simulink model "Drone_dynamic_controle_PID"  (R2024b)
settings: Solver=VariableStepAuto  StartTime=0.0  StopTime=20  RelTol=1e-3
values from neighbouring files (symbols this model uses):
  b = 4*1e-4    (= 0.0004)    [Drone_parameters.m]    (also in Quadcopter.m = 1e-06; drone_dynamics.m = 1e-06)
  g = 9.81    [Drone_parameters.m]    (also in Quadcopter.m; drone_dynamics.m)
  Ix = 0.02    [Drone_parameters.m]    (also in drone_dynamics.m)
  Iy = 0.02    [Drone_parameters.m]    (also in drone_dynamics.m)
  Iz = 0.04    [Drone_parameters.m]    (also in drone_dynamics.m)
  kf = T*0.7/w^2 * 0.8    (= 6.88114119063e-05)    [Drone_parameters.m]
  m = 1.2    [Drone_parameters.m]    (also in Quadcopter.m = 1; drone_dynamics.m)
  w_max = 2*3.14*n_max/60    (= 3061.60466667)    [Drone_parameters.m]
undefined symbols (not defined in the file or in its folder): a, balljoint_offset, k_cmd2rad, Kd_phi, Kd_psi, Kd_th, Kd_z, Ki_phi, Ki_psi, Ki_th, Ki_z, Kp_phi, Kp_psi, Kp_th, Kp_z, N_d, omega_max, omega_min, PID_LIMIT, PID_LIMIT_Z, s_max, s_min, SPEED_OFFSET, tau_m, tau_s, wmax
libraries: slpidlib x8
settings Model: Creator=lolme  LastModifiedBy=Rogul

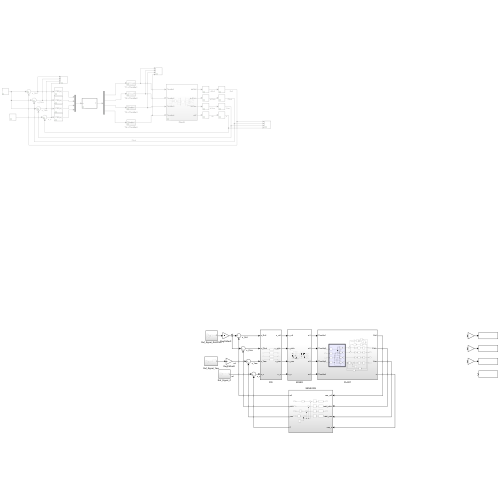
[thumbnail: Simulink's stored preview of the top-level diagram]
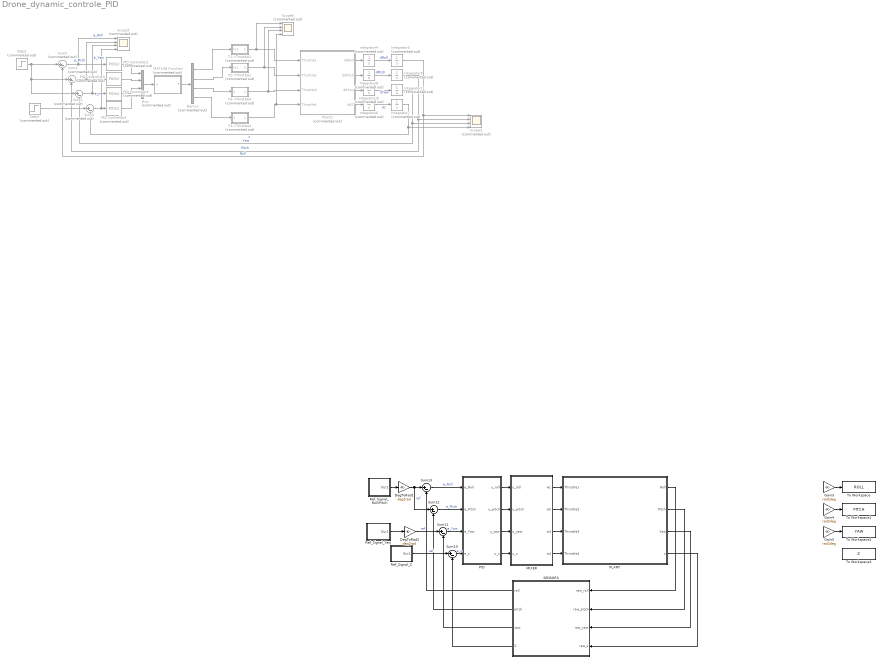
== system Drone_dynamic_controle_PID ==
  DegToRad1 : Gain  Gain=deg2rad
  DegToRad2 : Gain  Gain=deg2rad
  Demux : Demux  Commented=on
  Gain3 : Gain  Gain=rad2deg
  Gain4 : Gain  Gain=rad2deg
  Gain5 : Gain  Gain=rad2deg
  Integrator{4..11} (8 alike) : Integrator  Commented=on
  MATLAB Function : MATLAB Function  Commented=on  TreatAsAtomicUnit=on
  MIXER : Subsystem
  Mux : Mux  Commented=on
  PID : Subsystem
  PID Controller2 : slpidlib/PID Controller  Commented=on  Controller=PID  Form=Parallel  TimeDomain=Continuous-time  UseExternalTs=off  SampleTime=-1  IntegratorMethod=Forward Euler  FilterMethod=Forward Euler  ControllerParametersSource=internal  P=1.5  I=0.05  UseKiTs=off  D=0.3  UseExternalDerivativeSource=off  N=100  UseFilter=on  TunerSelectOption=Transfer Function Based (PID Tuner App)  InitialConditionSource=internal  InitialConditionForIntegrator=0  InitialConditionForFilter=0  DifferentiatorICPrevScaledInput=0  ExternalReset=none  TrackingMode=off  Kt=1  LimitOutput=off  SatLimitsSource=internal  UpperSaturationLimit=inf  LowerSaturationLimit=-inf  LinearizeAsGain=on  AntiWindupMode=none  Kb=1  LimitIntegrator=off  UpperIntegratorSaturationLimit=inf  LowerIntegratorSaturationLimit=-inf  POutMin=[]  POutMax=[]  IOutMin=[]  IOutMax=[]  DOutMin=[]  DOutMax=[]  NOutMin=[]  NOutMax=[]  SumOutMin=[]  SumOutMax=[]  SaturationOutMin=[]  SaturationOutMax=[]  PParamMin=[]  PParamMax=[]  IParamMin=[]  IParamMax=[]  DParamMin=[]  DParamMax=[]  NParamMin=[]  NParamMax=[]  KbParamMin=[]  KbParamMax=[]  KtParamMin=[]  KtParamMax=[]  KbOutMin=[]  KbOutMax=[]  KtOutMin=[]  KtOutMax=[]  IntegratorOutMin=[]  IntegratorOutMax=[]  FilterOutMin=[]  FilterOutMax=[]  SumI1OutMin=[]  SumI1OutMax=[]  SumI2OutMin=[]  SumI2OutMax=[]  SumI3OutMin=[]  SumI3OutMax=[]  SumI4OutMin=[]  SumI4OutMax=[]  SumDOutMin=[]  SumDOutMax=[]  DifferentiatorOutMin=[]  DifferentiatorOutMax=[]  FilterDiffOutCoefMin=[]  FilterDiffOutCoefMax=[]  ReciprocalOutMin=[]  ReciprocalOutMax=[]  SumDenOutMin=[]  SumDenOutMax=[]  SumNumOutMin=[]  SumNumOutMax=[]  DivideOutMin=[]  DivideOutMax=[]  UdiffTsProdOutMin=[]  UdiffTsProdOutMax=[]  NTsProdOutMin=[]  NTsProdOutMax=[]  UintegralTsProdOutMin=[]  UintegralTsProdOutMax=[]  UngainTsProdOutMin=[]  UngainTsProdOutMax=[]  ClampingZeroOutDataTypeStr=Inherit: Inherit via back propagation  ClampingZeroOutMin=[]  ClampingZeroOutMax=[]  FilterDenConstantOutDataTypeStr=Inherit: Inherit via back propagation  FilterDenConstantOutMin=[]  FilterDenConstantOutMax=[]  PCopyOutDataTypeStr=Inherit: Inherit via back propagation  PCopyOutMin=[]  PCopyOutMax=[]  NCopyOutDataTypeStr=Inherit: Inherit via back propagation  NCopyOutMin=[]  NCopyOutMax=[]  IntegratorContinuousStateAttributes=''  IntegratorStateMustResolveToSignalObject=off  IntegratorRTWStateStorageClass=Auto  FilterContinuousStateAttributes=''  FilterStateMustResolveToSignalObject=off  FilterRTWStateStorageClass=Auto  ParallelPVariant=InternalParameters  IdealPVariant=Disabled  IVariant=InternalParameters  DVariant=InternalParameters  IntegratorVariant=Continuous  SatVariant=Disabled  AWVariant=Passthrough  PCopyVariant=Disabled  TRVariant=Disabled  FdbkBlocksVariant=Forward  IdealPFdbkVariant=Disabled  SatFdbkVariant=Disabled  DerivativeFilterVariant=ContFilter  NVariant=InternalParameters  NCopyVariant=Disabled  FilterICVariant=InternalICsFilter  IntegratorICVariant=InternalICs  ExternalResetVariant=Disabled  TRSumVariant=Passthrough  SumFdbkVariant=Disabled  SumVariant=Sum_PID  TsampFilterVariant=InternalTs  TsampNgainVariant=Passthrough  TsampIntegralVariant=Disabled_SignalSpec  ExternalSaturationOutDataTypeStr=Inherit: Same as second input  DerivativeSourceVariant=ErrorSignal  PreIntVariant=InternalPreInt
  PID Controller3 : slpidlib/PID Controller  Commented=on  Controller=PID  Form=Parallel  TimeDomain=Continuous-time  UseExternalTs=off  SampleTime=-1  IntegratorMethod=Forward Euler  FilterMethod=Forward Euler  ControllerParametersSource=internal  P=1.5  I=0.05  UseKiTs=off  D=0.3  UseExternalDerivativeSource=off  N=100  UseFilter=on  TunerSelectOption=Transfer Function Based (PID Tuner App)  InitialConditionSource=internal  InitialConditionForIntegrator=0  InitialConditionForFilter=0  DifferentiatorICPrevScaledInput=0  ExternalReset=none  TrackingMode=off  Kt=1  LimitOutput=off  SatLimitsSource=internal  UpperSaturationLimit=inf  LowerSaturationLimit=-inf  LinearizeAsGain=on  AntiWindupMode=none  Kb=1  LimitIntegrator=off  UpperIntegratorSaturationLimit=inf  LowerIntegratorSaturationLimit=-inf  POutMin=[]  POutMax=[]  IOutMin=[]  IOutMax=[]  DOutMin=[]  DOutMax=[]  NOutMin=[]  NOutMax=[]  SumOutMin=[]  SumOutMax=[]  SaturationOutMin=[]  SaturationOutMax=[]  PParamMin=[]  PParamMax=[]  IParamMin=[]  IParamMax=[]  DParamMin=[]  DParamMax=[]  NParamMin=[]  NParamMax=[]  KbParamMin=[]  KbParamMax=[]  KtParamMin=[]  KtParamMax=[]  KbOutMin=[]  KbOutMax=[]  KtOutMin=[]  KtOutMax=[]  IntegratorOutMin=[]  IntegratorOutMax=[]  FilterOutMin=[]  FilterOutMax=[]  SumI1OutMin=[]  SumI1OutMax=[]  SumI2OutMin=[]  SumI2OutMax=[]  SumI3OutMin=[]  SumI3OutMax=[]  SumI4OutMin=[]  SumI4OutMax=[]  SumDOutMin=[]  SumDOutMax=[]  DifferentiatorOutMin=[]  DifferentiatorOutMax=[]  FilterDiffOutCoefMin=[]  FilterDiffOutCoefMax=[]  ReciprocalOutMin=[]  ReciprocalOutMax=[]  SumDenOutMin=[]  SumDenOutMax=[]  SumNumOutMin=[]  SumNumOutMax=[]  DivideOutMin=[]  DivideOutMax=[]  UdiffTsProdOutMin=[]  UdiffTsProdOutMax=[]  NTsProdOutMin=[]  NTsProdOutMax=[]  UintegralTsProdOutMin=[]  UintegralTsProdOutMax=[]  UngainTsProdOutMin=[]  UngainTsProdOutMax=[]  ClampingZeroOutDataTypeStr=Inherit: Inherit via back propagation  ClampingZeroOutMin=[]  ClampingZeroOutMax=[]  FilterDenConstantOutDataTypeStr=Inherit: Inherit via back propagation  FilterDenConstantOutMin=[]  FilterDenConstantOutMax=[]  PCopyOutDataTypeStr=Inherit: Inherit via back propagation  PCopyOutMin=[]  PCopyOutMax=[]  NCopyOutDataTypeStr=Inherit: Inherit via back propagation  NCopyOutMin=[]  NCopyOutMax=[]  IntegratorContinuousStateAttributes=''  IntegratorStateMustResolveToSignalObject=off  IntegratorRTWStateStorageClass=Auto  FilterContinuousStateAttributes=''  FilterStateMustResolveToSignalObject=off  FilterRTWStateStorageClass=Auto  ParallelPVariant=InternalParameters  IdealPVariant=Disabled  IVariant=InternalParameters  DVariant=InternalParameters  IntegratorVariant=Continuous  SatVariant=Disabled  AWVariant=Passthrough  PCopyVariant=Disabled  TRVariant=Disabled  FdbkBlocksVariant=Forward  IdealPFdbkVariant=Disabled  SatFdbkVariant=Disabled  DerivativeFilterVariant=ContFilter  NVariant=InternalParameters  NCopyVariant=Disabled  FilterICVariant=InternalICsFilter  IntegratorICVariant=InternalICs  ExternalResetVariant=Disabled  TRSumVariant=Passthrough  SumFdbkVariant=Disabled  SumVariant=Sum_PID  TsampFilterVariant=InternalTs  TsampNgainVariant=Passthrough  TsampIntegralVariant=Disabled_SignalSpec  ExternalSaturationOutDataTypeStr=Inherit: Same as second input  DerivativeSourceVariant=ErrorSignal  PreIntVariant=InternalPreInt
  PID Controller4 : slpidlib/PID Controller  Commented=on  Controller=PID  Form=Parallel  TimeDomain=Continuous-time  UseExternalTs=off  SampleTime=-1  IntegratorMethod=Forward Euler  FilterMethod=Forward Euler  ControllerParametersSource=internal  P=1.5  I=0.05  UseKiTs=off  D=0.3  UseExternalDerivativeSource=off  N=100  UseFilter=on  TunerSelectOption=Transfer Function Based (PID Tuner App)  InitialConditionSource=internal  InitialConditionForIntegrator=0  InitialConditionForFilter=0  DifferentiatorICPrevScaledInput=0  ExternalReset=none  TrackingMode=off  Kt=1  LimitOutput=off  SatLimitsSource=internal  UpperSaturationLimit=inf  LowerSaturationLimit=-inf  LinearizeAsGain=on  AntiWindupMode=none  Kb=1  LimitIntegrator=off  UpperIntegratorSaturationLimit=inf  LowerIntegratorSaturationLimit=-inf  POutMin=[]  POutMax=[]  IOutMin=[]  IOutMax=[]  DOutMin=[]  DOutMax=[]  NOutMin=[]  NOutMax=[]  SumOutMin=[]  SumOutMax=[]  SaturationOutMin=[]  SaturationOutMax=[]  PParamMin=[]  PParamMax=[]  IParamMin=[]  IParamMax=[]  DParamMin=[]  DParamMax=[]  NParamMin=[]  NParamMax=[]  KbParamMin=[]  KbParamMax=[]  KtParamMin=[]  KtParamMax=[]  KbOutMin=[]  KbOutMax=[]  KtOutMin=[]  KtOutMax=[]  IntegratorOutMin=[]  IntegratorOutMax=[]  FilterOutMin=[]  FilterOutMax=[]  SumI1OutMin=[]  SumI1OutMax=[]  SumI2OutMin=[]  SumI2OutMax=[]  SumI3OutMin=[]  SumI3OutMax=[]  SumI4OutMin=[]  SumI4OutMax=[]  SumDOutMin=[]  SumDOutMax=[]  DifferentiatorOutMin=[]  DifferentiatorOutMax=[]  FilterDiffOutCoefMin=[]  FilterDiffOutCoefMax=[]  ReciprocalOutMin=[]  ReciprocalOutMax=[]  SumDenOutMin=[]  SumDenOutMax=[]  SumNumOutMin=[]  SumNumOutMax=[]  DivideOutMin=[]  DivideOutMax=[]  UdiffTsProdOutMin=[]  UdiffTsProdOutMax=[]  NTsProdOutMin=[]  NTsProdOutMax=[]  UintegralTsProdOutMin=[]  UintegralTsProdOutMax=[]  UngainTsProdOutMin=[]  UngainTsProdOutMax=[]  ClampingZeroOutDataTypeStr=Inherit: Inherit via back propagation  ClampingZeroOutMin=[]  ClampingZeroOutMax=[]  FilterDenConstantOutDataTypeStr=Inherit: Inherit via back propagation  FilterDenConstantOutMin=[]  FilterDenConstantOutMax=[]  PCopyOutDataTypeStr=Inherit: Inherit via back propagation  PCopyOutMin=[]  PCopyOutMax=[]  NCopyOutDataTypeStr=Inherit: Inherit via back propagation  NCopyOutMin=[]  NCopyOutMax=[]  IntegratorContinuousStateAttributes=''  IntegratorStateMustResolveToSignalObject=off  IntegratorRTWStateStorageClass=Auto  FilterContinuousStateAttributes=''  FilterStateMustResolveToSignalObject=off  FilterRTWStateStorageClass=Auto  ParallelPVariant=InternalParameters  IdealPVariant=Disabled  IVariant=InternalParameters  DVariant=InternalParameters  IntegratorVariant=Continuous  SatVariant=Disabled  AWVariant=Passthrough  PCopyVariant=Disabled  TRVariant=Disabled  FdbkBlocksVariant=Forward  IdealPFdbkVariant=Disabled  SatFdbkVariant=Disabled  DerivativeFilterVariant=ContFilter  NVariant=InternalParameters  NCopyVariant=Disabled  FilterICVariant=InternalICsFilter  IntegratorICVariant=InternalICs  ExternalResetVariant=Disabled  TRSumVariant=Passthrough  SumFdbkVariant=Disabled  SumVariant=Sum_PID  TsampFilterVariant=InternalTs  TsampNgainVariant=Passthrough  TsampIntegralVariant=Disabled_SignalSpec  ExternalSaturationOutDataTypeStr=Inherit: Same as second input  DerivativeSourceVariant=ErrorSignal  PreIntVariant=InternalPreInt
  PID Controller5 : slpidlib/PID Controller  Commented=on  Controller=PID  Form=Parallel  TimeDomain=Continuous-time  UseExternalTs=off  SampleTime=-1  IntegratorMethod=Forward Euler  FilterMethod=Forward Euler  ControllerParametersSource=internal  P=20  I=5  UseKiTs=off  D=10  UseExternalDerivativeSource=off  N=100  UseFilter=on  TunerSelectOption=Transfer Function Based (PID Tuner App)  InitialConditionSource=internal  InitialConditionForIntegrator=0  InitialConditionForFilter=0  DifferentiatorICPrevScaledInput=0  ExternalReset=none  TrackingMode=off  Kt=1  LimitOutput=off  SatLimitsSource=internal  UpperSaturationLimit=inf  LowerSaturationLimit=-inf  LinearizeAsGain=on  AntiWindupMode=none  Kb=1  LimitIntegrator=off  UpperIntegratorSaturationLimit=inf  LowerIntegratorSaturationLimit=-inf  POutMin=[]  POutMax=[]  IOutMin=[]  IOutMax=[]  DOutMin=[]  DOutMax=[]  NOutMin=[]  NOutMax=[]  SumOutMin=[]  SumOutMax=[]  SaturationOutMin=[]  SaturationOutMax=[]  PParamMin=[]  PParamMax=[]  IParamMin=[]  IParamMax=[]  DParamMin=[]  DParamMax=[]  NParamMin=[]  NParamMax=[]  KbParamMin=[]  KbParamMax=[]  KtParamMin=[]  KtParamMax=[]  KbOutMin=[]  KbOutMax=[]  KtOutMin=[]  KtOutMax=[]  IntegratorOutMin=[]  IntegratorOutMax=[]  FilterOutMin=[]  FilterOutMax=[]  SumI1OutMin=[]  SumI1OutMax=[]  SumI2OutMin=[]  SumI2OutMax=[]  SumI3OutMin=[]  SumI3OutMax=[]  SumI4OutMin=[]  SumI4OutMax=[]  SumDOutMin=[]  SumDOutMax=[]  DifferentiatorOutMin=[]  DifferentiatorOutMax=[]  FilterDiffOutCoefMin=[]  FilterDiffOutCoefMax=[]  ReciprocalOutMin=[]  ReciprocalOutMax=[]  SumDenOutMin=[]  SumDenOutMax=[]  SumNumOutMin=[]  SumNumOutMax=[]  DivideOutMin=[]  DivideOutMax=[]  UdiffTsProdOutMin=[]  UdiffTsProdOutMax=[]  NTsProdOutMin=[]  NTsProdOutMax=[]  UintegralTsProdOutMin=[]  UintegralTsProdOutMax=[]  UngainTsProdOutMin=[]  UngainTsProdOutMax=[]  ClampingZeroOutDataTypeStr=Inherit: Inherit via back propagation  ClampingZeroOutMin=[]  ClampingZeroOutMax=[]  FilterDenConstantOutDataTypeStr=Inherit: Inherit via back propagation  FilterDenConstantOutMin=[]  FilterDenConstantOutMax=[]  PCopyOutDataTypeStr=Inherit: Inherit via back propagation  PCopyOutMin=[]  PCopyOutMax=[]  NCopyOutDataTypeStr=Inherit: Inherit via back propagation  NCopyOutMin=[]  NCopyOutMax=[]  IntegratorContinuousStateAttributes=''  IntegratorStateMustResolveToSignalObject=off  IntegratorRTWStateStorageClass=Auto  FilterContinuousStateAttributes=''  FilterStateMustResolveToSignalObject=off  FilterRTWStateStorageClass=Auto  ParallelPVariant=InternalParameters  IdealPVariant=Disabled  IVariant=InternalParameters  DVariant=InternalParameters  IntegratorVariant=Continuous  SatVariant=Disabled  AWVariant=Passthrough  PCopyVariant=Disabled  TRVariant=Disabled  FdbkBlocksVariant=Forward  IdealPFdbkVariant=Disabled  SatFdbkVariant=Disabled  DerivativeFilterVariant=ContFilter  NVariant=InternalParameters  NCopyVariant=Disabled  FilterICVariant=InternalICsFilter  IntegratorICVariant=InternalICs  ExternalResetVariant=Disabled  TRSumVariant=Passthrough  SumFdbkVariant=Disabled  SumVariant=Sum_PID  TsampFilterVariant=InternalTs  TsampNgainVariant=Passthrough  TsampIntegralVariant=Disabled_SignalSpec  ExternalSaturationOutDataTypeStr=Inherit: Same as second input  DerivativeSourceVariant=ErrorSignal  PreIntVariant=InternalPreInt
  PLANT : Subsystem
  Plant2 : Subsystem  Commented=on
  Ref_Signal_Roll/Pitch : Subsystem
  Ref_Signal_Yaw : Subsystem
  Ref_Signal_Z : Subsystem
  SENSORS : Subsystem
  Scope3 : Scope  Commented=on  NumInputPorts=4
  Scope5 : Scope  Commented=on  NumInputPorts=4
  Scope6 : Scope  Commented=on  NumInputPorts=4
  Step2 : Step  Commented=on  Time=5  Before=20  After=0  SampleTime=0
  Step3 : Step  Commented=on  Time=5  Before=10  After=20  SampleTime=0
  Sum{10..13} (4 alike) : Sum  Inputs=|+-
  Sum{2..5} (4 alike) : Sum  Commented=on  Inputs=|+-
  T1->Throttle1 : Subsystem  Commented=on
  T2->Throttle2 : Subsystem  Commented=on
  T3->Throttle3 : Subsystem  Commented=on
  T4->Throttle4 : Subsystem  Commented=on
  To Workspace : ToWorkspace  VariableName=ROLL  SaveFormat=Timeseries  SampleTime=0.01
      settings: Save2DSignal=2-D array (concatenate along first dimension)
  To Workspace1 : ToWorkspace  VariableName=PITCH  SaveFormat=Timeseries  SampleTime=0.01
      settings: Save2DSignal=2-D array (concatenate along first dimension)
  To Workspace2 : ToWorkspace  VariableName=YAW  SaveFormat=Timeseries  SampleTime=0.01
      settings: Save2DSignal=2-D array (concatenate along first dimension)
  To Workspace3 : ToWorkspace  VariableName=Z  SaveFormat=Timeseries  SampleTime=0.01
      settings: Save2DSignal=2-D array (concatenate along first dimension)
  wires:
  Integrator7/1 -> Scope3/4, Sum2/2  "z"
  Integrator4/1 -> Integrator5/1  "dRoll"
  Plant2/1(ddRoll) -> Integrator4/1
  Integrator6/1 -> Integrator7/1  "dz"
  Integrator5/1 -> Scope3/1, Sum5/2  "Roll"
  Plant2/4(ddZ) -> Integrator6/1
  Integrator9/1 -> Scope3/2, Sum4/2  "Pitch"
  Plant2/2(ddPitch) -> Integrator8/1
  Integrator8/1 -> Integrator9/1  "dPitch"
  Plant2/3(ddYaw) -> Integrator10/1
  Integrator10/1 -> Integrator11/1  "dYaw"
  Integrator11/1 -> Scope3/3, Sum3/2  "Yaw"
  Sum2/1 -> Scope5/4, PID Controller5/1  "e_z"
  Sum3/1 -> Scope5/3, PID Controller4/1  "e_Yaw"
  Sum4/1 -> Scope5/2, PID Controller3/1  "e_Pitch"
  Sum5/1 -> Scope5/1, PID Controller2/1  "e_Roll"
  Step2/1 -> Sum3/1, Sum4/1, Sum5/1
  Step3/1 -> Sum2/1
  PID Controller2/1 -> Mux/1
  PID Controller3/1 -> Mux/2
  PID Controller4/1 -> Mux/3
  PID Controller5/1 -> Mux/4
  Mux/1 -> MATLAB Function/1(u)
  MATLAB Function/1(T) -> Demux/1
  Demux/1 -> T1->Throttle1/1(In1)
  T2->Throttle2/1(1) -> Scope6/2, Plant2/2(Throttle2)
  Demux/2 -> T2->Throttle2/1(In1)
  T3->Throttle3/1(Throttle1) -> Scope6/3, Plant2/3(Throttle3)
  Demux/3 -> T3->Throttle3/1(In1)
  T4->Throttle4/1(Throttle1) -> Scope6/4, Plant2/4(Throttle4)
  Demux/4 -> T4->Throttle4/1(In1)
  T1->Throttle1/1(1) -> Scope6/1, Plant2/1(Throttle1)
  Ref_Signal_Roll/Pitch/1(Out1) -> DegToRad1/1
  Ref_Signal_Yaw/1(Out1) -> DegToRad2/1
  Ref_Signal_Z/1(Out1) -> Sum10/1  "ref"
  DegToRad1/1 -> Sum13/1, Sum12/1  "ref"
  DegToRad2/1 -> Sum11/1  "ref"
  MIXER/1(w1) -> PLANT/1(Throttle1)
  MIXER/2(w2) -> PLANT/2(Throttle2)
  MIXER/3(w3) -> PLANT/3(Throttle3)
  MIXER/4(w4) -> PLANT/4(Throttle4)
  Gain3/1 -> To Workspace/1
  Gain4/1 -> To Workspace1/1
  Gain5/1 -> To Workspace2/1
  Sum13/1 -> PID/1(e_Roll)  "e_Roll"
  Sum12/1 -> PID/2(e_Pitch)  "e_Pitch"
  Sum11/1 -> PID/3(e_Yaw)  "e_Yaw"
  Sum10/1 -> PID/4(e_z)  "e_z"
  PID/1(u_roll) -> MIXER/1(u_roll)
  PID/2(u_pitch) -> MIXER/2(u_pitch)
  PID/3(u_yaw) -> MIXER/3(u_yaw)
  PID/4(u_z) -> MIXER/4(u_z)
  PLANT/1(Roll) -> SENSORS/1(raw_roll)
  PLANT/2(Pitch) -> SENSORS/2(raw_pitch)
  PLANT/3(Yaw) -> SENSORS/3(raw_yaw)
  PLANT/4(z) -> SENSORS/4(raw_z)
  SENSORS/1(roll) -> Sum13/2
  SENSORS/2(pitch) -> Sum12/2
  SENSORS/4(Z) -> Sum10/2
  SENSORS/3(yaw) -> Sum11/2

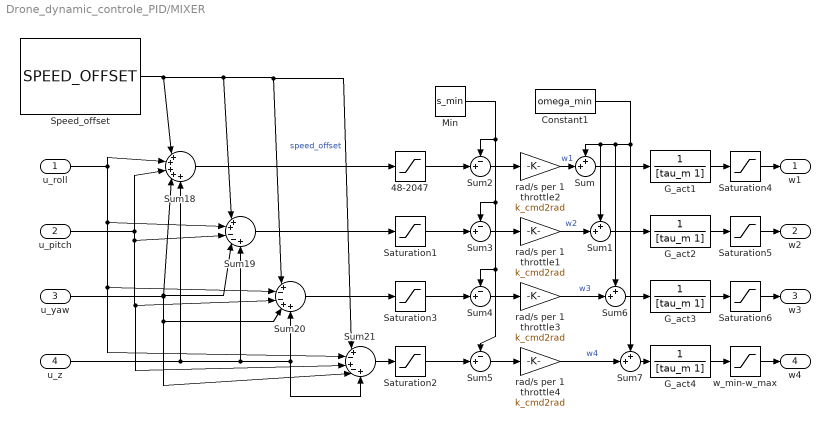
== system Drone_dynamic_controle_PID/MIXER ==
  u_roll : Inport
  u_pitch : Inport  Port=2
  u_yaw : Inport  Port=3
  u_z : Inport  Port=4
  48-2047 : Saturate  UpperLimit=s_max  LowerLimit=s_min
  Constant1 : Constant  Value=omega_min
  G_act{1..4} (4 alike) : TransferFcn  Denominator=[tau_m 1]
  Min : Constant  Value=s_min
  Saturation1 : Saturate  UpperLimit=s_max  LowerLimit=s_min
  Saturation2 : Saturate  UpperLimit=s_max  LowerLimit=s_min
  Saturation3 : Saturate  UpperLimit=s_max  LowerLimit=s_min
  Saturation4 : Saturate  UpperLimit=omega_max  LowerLimit=omega_min
  Saturation5 : Saturate  UpperLimit=omega_max  LowerLimit=omega_min
  Saturation6 : Saturate  UpperLimit=omega_max  LowerLimit=omega_min
  Speed_offset : Constant  Value=SPEED_OFFSET
  Sum{,1,6..7} (4 alike) : Sum  Inputs=++|
  Sum18 : Sum  Inputs=|+++++
  Sum19 : Sum  Inputs=|++--+
  Sum{2..5} (4 alike) : Sum  Inputs=-+|
  Sum20 : Sum  Inputs=|+--++
  Sum21 : Sum  Inputs=|+-+-+
  rad/s per 1 throttle{1..4} (4 alike) : Gain  Gain=k_cmd2rad
  w_min-w_max : Saturate  UpperLimit=omega_max  LowerLimit=omega_min
  w1 : Outport
  w2 : Outport  Port=2
  w3 : Outport  Port=3
  w4 : Outport  Port=4
  wires:
  Sum21/1 -> Saturation2/1
  u_pitch/1 -> Sum21/3, Sum20/3, Sum19/3, Sum18/3
  u_z/1 -> Sum18/5, Sum19/5, Sum20/5, Sum21/5
  Speed_offset/1 -> Sum21/1, Sum20/1, Sum19/1, Sum18/1  "speed_offset"
  u_roll/1 -> Sum21/2, Sum20/2, Sum19/2, Sum18/2
  u_yaw/1 -> Sum18/4, Sum19/4, Sum20/4, Sum21/4
  Sum20/1 -> Saturation3/1
  Sum18/1 -> 48-2047/1
  Sum19/1 -> Saturation1/1
  48-2047/1 -> Sum2/2
  Constant1/1 -> Sum/1, Sum1/1, Sum6/1, Sum7/1
  Sum/1 -> G_act1/1
  Saturation1/1 -> Sum3/2
  rad/s per 1 throttle1/1 -> Sum1/2  "w2"
  Saturation2/1 -> Sum5/2
  rad/s per 1 throttle4/1 -> Sum7/2  "w4"
  Sum2/1 -> rad/s per 1 throttle2/1
  Sum4/1 -> rad/s per 1 throttle3/1
  Sum5/1 -> rad/s per 1 throttle4/1
  rad/s per 1 throttle2/1 -> Sum/2  "w1"
  rad/s per 1 throttle3/1 -> Sum6/2  "w3"
  G_act3/1 -> Saturation6/1
  G_act1/1 -> Saturation4/1
  Saturation3/1 -> Sum4/2
  Min/1 -> Sum3/1, Sum4/1, Sum5/1, Sum2/1
  Sum7/1 -> G_act4/1
  G_act2/1 -> Saturation5/1
  Sum3/1 -> rad/s per 1 throttle1/1
  Sum1/1 -> G_act2/1
  G_act4/1 -> w_min-w_max/1
  Sum6/1 -> G_act3/1
  w_min-w_max/1 -> w4/1
  Saturation4/1 -> w1/1
  Saturation5/1 -> w2/1
  Saturation6/1 -> w3/1

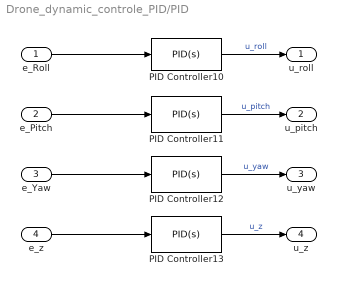
== system Drone_dynamic_controle_PID/PID ==
  e_Roll : Inport
  e_Pitch : Inport  Port=2
  e_Yaw : Inport  Port=3
  e_z : Inport  Port=4
  PID Controller10 : slpidlib/PID Controller  Controller=PID  Form=Parallel  TimeDomain=Continuous-time  UseExternalTs=off  SampleTime=0.01  IntegratorMethod=Trapezoidal  FilterMethod=Trapezoidal  ControllerParametersSource=internal  P=Kp_phi  I=Ki_phi  UseKiTs=off  D=Kd_phi  UseExternalDerivativeSource=off  N=N_d  UseFilter=on  TunerSelectOption=Transfer Function Based (PID Tuner App)  InitialConditionSource=internal  InitialConditionForIntegrator=0  InitialConditionForFilter=0  DifferentiatorICPrevScaledInput=0  ExternalReset=none  TrackingMode=off  Kt=1  LimitOutput=on  SatLimitsSource=internal  UpperSaturationLimit=PID_LIMIT  LowerSaturationLimit=-PID_LIMIT  LinearizeAsGain=on  AntiWindupMode=clamping  Kb=1  LimitIntegrator=off  UpperIntegratorSaturationLimit=inf  LowerIntegratorSaturationLimit=-inf  POutMin=[]  POutMax=[]  IOutMin=[]  IOutMax=[]  DOutMin=[]  DOutMax=[]  NOutMin=[]  NOutMax=[]  SumOutMin=[]  SumOutMax=[]  SaturationOutMin=[]  SaturationOutMax=[]  PParamMin=[]  PParamMax=[]  IParamMin=[]  IParamMax=[]  DParamMin=[]  DParamMax=[]  NParamMin=[]  NParamMax=[]  KbParamMin=[]  KbParamMax=[]  KtParamMin=[]  KtParamMax=[]  KbOutMin=[]  KbOutMax=[]  KtOutMin=[]  KtOutMax=[]  IntegratorOutMin=[]  IntegratorOutMax=[]  FilterOutMin=[]  FilterOutMax=[]  SumI1OutMin=[]  SumI1OutMax=[]  SumI2OutMin=[]  SumI2OutMax=[]  SumI3OutMin=[]  SumI3OutMax=[]  SumI4OutMin=[]  SumI4OutMax=[]  SumDOutMin=[]  SumDOutMax=[]  DifferentiatorOutMin=[]  DifferentiatorOutMax=[]  FilterDiffOutCoefMin=[]  FilterDiffOutCoefMax=[]  ReciprocalOutMin=[]  ReciprocalOutMax=[]  SumDenOutMin=[]  SumDenOutMax=[]  SumNumOutMin=[]  SumNumOutMax=[]  DivideOutMin=[]  DivideOutMax=[]  UdiffTsProdOutMin=[]  UdiffTsProdOutMax=[]  NTsProdOutMin=[]  NTsProdOutMax=[]  UintegralTsProdOutMin=[]  UintegralTsProdOutMax=[]  UngainTsProdOutMin=[]  UngainTsProdOutMax=[]  ClampingZeroOutDataTypeStr=Inherit: Inherit via back propagation  ClampingZeroOutMin=[]  ClampingZeroOutMax=[]  FilterDenConstantOutDataTypeStr=Inherit: Inherit via back propagation  FilterDenConstantOutMin=[]  FilterDenConstantOutMax=[]  PCopyOutDataTypeStr=Inherit: Inherit via back propagation  PCopyOutMin=[]  PCopyOutMax=[]  NCopyOutDataTypeStr=Inherit: Inherit via back propagation  NCopyOutMin=[]  NCopyOutMax=[]  IntegratorContinuousStateAttributes=''  IntegratorStateMustResolveToSignalObject=off  IntegratorRTWStateStorageClass=Auto  FilterContinuousStateAttributes=''  FilterStateMustResolveToSignalObject=off  FilterRTWStateStorageClass=Auto  ParallelPVariant=InternalParameters  IdealPVariant=Disabled  IVariant=InternalParameters  DVariant=InternalParameters  IntegratorVariant=Continuous  SatVariant=Enabled  AWVariant=ContClampingParallel  PCopyVariant=Disabled  TRVariant=Disabled  FdbkBlocksVariant=Forward  IdealPFdbkVariant=Disabled  SatFdbkVariant=Disabled  DerivativeFilterVariant=ContFilter  NVariant=InternalParameters  NCopyVariant=Disabled  FilterICVariant=InternalICsFilter  IntegratorICVariant=InternalICs  ExternalResetVariant=Disabled  TRSumVariant=Passthrough  SumFdbkVariant=Disabled  SumVariant=Sum_PID  TsampFilterVariant=InternalTs  TsampNgainVariant=Passthrough  TsampIntegralVariant=Disabled_SignalSpec  ExternalSaturationOutDataTypeStr=Inherit: Same as second input  DerivativeSourceVariant=ErrorSignal  PreIntVariant=InternalPreInt
  PID Controller11 : slpidlib/PID Controller  Controller=PID  Form=Parallel  TimeDomain=Continuous-time  UseExternalTs=off  SampleTime=0.01  IntegratorMethod=Trapezoidal  FilterMethod=Trapezoidal  ControllerParametersSource=internal  P=Kp_th  I=Ki_th  UseKiTs=off  D=Kd_th  UseExternalDerivativeSource=off  N=N_d  UseFilter=on  TunerSelectOption=Transfer Function Based (PID Tuner App)  InitialConditionSource=internal  InitialConditionForIntegrator=0  InitialConditionForFilter=0  DifferentiatorICPrevScaledInput=0  ExternalReset=none  TrackingMode=off  Kt=1  LimitOutput=on  SatLimitsSource=internal  UpperSaturationLimit=PID_LIMIT  LowerSaturationLimit=-PID_LIMIT  LinearizeAsGain=on  AntiWindupMode=clamping  Kb=1  LimitIntegrator=off  UpperIntegratorSaturationLimit=inf  LowerIntegratorSaturationLimit=-inf  POutMin=[]  POutMax=[]  IOutMin=[]  IOutMax=[]  DOutMin=[]  DOutMax=[]  NOutMin=[]  NOutMax=[]  SumOutMin=[]  SumOutMax=[]  SaturationOutMin=[]  SaturationOutMax=[]  PParamMin=[]  PParamMax=[]  IParamMin=[]  IParamMax=[]  DParamMin=[]  DParamMax=[]  NParamMin=[]  NParamMax=[]  KbParamMin=[]  KbParamMax=[]  KtParamMin=[]  KtParamMax=[]  KbOutMin=[]  KbOutMax=[]  KtOutMin=[]  KtOutMax=[]  IntegratorOutMin=[]  IntegratorOutMax=[]  FilterOutMin=[]  FilterOutMax=[]  SumI1OutMin=[]  SumI1OutMax=[]  SumI2OutMin=[]  SumI2OutMax=[]  SumI3OutMin=[]  SumI3OutMax=[]  SumI4OutMin=[]  SumI4OutMax=[]  SumDOutMin=[]  SumDOutMax=[]  DifferentiatorOutMin=[]  DifferentiatorOutMax=[]  FilterDiffOutCoefMin=[]  FilterDiffOutCoefMax=[]  ReciprocalOutMin=[]  ReciprocalOutMax=[]  SumDenOutMin=[]  SumDenOutMax=[]  SumNumOutMin=[]  SumNumOutMax=[]  DivideOutMin=[]  DivideOutMax=[]  UdiffTsProdOutMin=[]  UdiffTsProdOutMax=[]  NTsProdOutMin=[]  NTsProdOutMax=[]  UintegralTsProdOutMin=[]  UintegralTsProdOutMax=[]  UngainTsProdOutMin=[]  UngainTsProdOutMax=[]  ClampingZeroOutDataTypeStr=Inherit: Inherit via back propagation  ClampingZeroOutMin=[]  ClampingZeroOutMax=[]  FilterDenConstantOutDataTypeStr=Inherit: Inherit via back propagation  FilterDenConstantOutMin=[]  FilterDenConstantOutMax=[]  PCopyOutDataTypeStr=Inherit: Inherit via back propagation  PCopyOutMin=[]  PCopyOutMax=[]  NCopyOutDataTypeStr=Inherit: Inherit via back propagation  NCopyOutMin=[]  NCopyOutMax=[]  IntegratorContinuousStateAttributes=''  IntegratorStateMustResolveToSignalObject=off  IntegratorRTWStateStorageClass=Auto  FilterContinuousStateAttributes=''  FilterStateMustResolveToSignalObject=off  FilterRTWStateStorageClass=Auto  ParallelPVariant=InternalParameters  IdealPVariant=Disabled  IVariant=InternalParameters  DVariant=InternalParameters  IntegratorVariant=Continuous  SatVariant=Enabled  AWVariant=ContClampingParallel  PCopyVariant=Disabled  TRVariant=Disabled  FdbkBlocksVariant=Forward  IdealPFdbkVariant=Disabled  SatFdbkVariant=Disabled  DerivativeFilterVariant=ContFilter  NVariant=InternalParameters  NCopyVariant=Disabled  FilterICVariant=InternalICsFilter  IntegratorICVariant=InternalICs  ExternalResetVariant=Disabled  TRSumVariant=Passthrough  SumFdbkVariant=Disabled  SumVariant=Sum_PID  TsampFilterVariant=InternalTs  TsampNgainVariant=Passthrough  TsampIntegralVariant=Disabled_SignalSpec  ExternalSaturationOutDataTypeStr=Inherit: Same as second input  DerivativeSourceVariant=ErrorSignal  PreIntVariant=InternalPreInt
  PID Controller12 : slpidlib/PID Controller  Controller=PID  Form=Parallel  TimeDomain=Continuous-time  UseExternalTs=off  SampleTime=0.01  IntegratorMethod=Trapezoidal  FilterMethod=Trapezoidal  ControllerParametersSource=internal  P=Kp_psi  I=Ki_psi  UseKiTs=off  D=Kd_psi  UseExternalDerivativeSource=off  N=N_d  UseFilter=on  TunerSelectOption=Transfer Function Based (PID Tuner App)  InitialConditionSource=internal  InitialConditionForIntegrator=0  InitialConditionForFilter=0  DifferentiatorICPrevScaledInput=0  ExternalReset=none  TrackingMode=off  Kt=1  LimitOutput=on  SatLimitsSource=internal  UpperSaturationLimit=PID_LIMIT  LowerSaturationLimit=-PID_LIMIT  LinearizeAsGain=on  AntiWindupMode=clamping  Kb=1  LimitIntegrator=off  UpperIntegratorSaturationLimit=inf  LowerIntegratorSaturationLimit=-inf  POutMin=[]  POutMax=[]  IOutMin=[]  IOutMax=[]  DOutMin=[]  DOutMax=[]  NOutMin=[]  NOutMax=[]  SumOutMin=[]  SumOutMax=[]  SaturationOutMin=[]  SaturationOutMax=[]  PParamMin=[]  PParamMax=[]  IParamMin=[]  IParamMax=[]  DParamMin=[]  DParamMax=[]  NParamMin=[]  NParamMax=[]  KbParamMin=[]  KbParamMax=[]  KtParamMin=[]  KtParamMax=[]  KbOutMin=[]  KbOutMax=[]  KtOutMin=[]  KtOutMax=[]  IntegratorOutMin=[]  IntegratorOutMax=[]  FilterOutMin=[]  FilterOutMax=[]  SumI1OutMin=[]  SumI1OutMax=[]  SumI2OutMin=[]  SumI2OutMax=[]  SumI3OutMin=[]  SumI3OutMax=[]  SumI4OutMin=[]  SumI4OutMax=[]  SumDOutMin=[]  SumDOutMax=[]  DifferentiatorOutMin=[]  DifferentiatorOutMax=[]  FilterDiffOutCoefMin=[]  FilterDiffOutCoefMax=[]  ReciprocalOutMin=[]  ReciprocalOutMax=[]  SumDenOutMin=[]  SumDenOutMax=[]  SumNumOutMin=[]  SumNumOutMax=[]  DivideOutMin=[]  DivideOutMax=[]  UdiffTsProdOutMin=[]  UdiffTsProdOutMax=[]  NTsProdOutMin=[]  NTsProdOutMax=[]  UintegralTsProdOutMin=[]  UintegralTsProdOutMax=[]  UngainTsProdOutMin=[]  UngainTsProdOutMax=[]  ClampingZeroOutDataTypeStr=Inherit: Inherit via back propagation  ClampingZeroOutMin=[]  ClampingZeroOutMax=[]  FilterDenConstantOutDataTypeStr=Inherit: Inherit via back propagation  FilterDenConstantOutMin=[]  FilterDenConstantOutMax=[]  PCopyOutDataTypeStr=Inherit: Inherit via back propagation  PCopyOutMin=[]  PCopyOutMax=[]  NCopyOutDataTypeStr=Inherit: Inherit via back propagation  NCopyOutMin=[]  NCopyOutMax=[]  IntegratorContinuousStateAttributes=''  IntegratorStateMustResolveToSignalObject=off  IntegratorRTWStateStorageClass=Auto  FilterContinuousStateAttributes=''  FilterStateMustResolveToSignalObject=off  FilterRTWStateStorageClass=Auto  ParallelPVariant=InternalParameters  IdealPVariant=Disabled  IVariant=InternalParameters  DVariant=InternalParameters  IntegratorVariant=Continuous  SatVariant=Enabled  AWVariant=ContClampingParallel  PCopyVariant=Disabled  TRVariant=Disabled  FdbkBlocksVariant=Forward  IdealPFdbkVariant=Disabled  SatFdbkVariant=Disabled  DerivativeFilterVariant=ContFilter  NVariant=InternalParameters  NCopyVariant=Disabled  FilterICVariant=InternalICsFilter  IntegratorICVariant=InternalICs  ExternalResetVariant=Disabled  TRSumVariant=Passthrough  SumFdbkVariant=Disabled  SumVariant=Sum_PID  TsampFilterVariant=InternalTs  TsampNgainVariant=Passthrough  TsampIntegralVariant=Disabled_SignalSpec  ExternalSaturationOutDataTypeStr=Inherit: Same as second input  DerivativeSourceVariant=ErrorSignal  PreIntVariant=InternalPreInt
  PID Controller13 : slpidlib/PID Controller  Controller=PID  Form=Parallel  TimeDomain=Continuous-time  UseExternalTs=off  SampleTime=0.01  IntegratorMethod=Trapezoidal  FilterMethod=Trapezoidal  ControllerParametersSource=internal  P=Kp_z  I=Ki_z  UseKiTs=off  D=Kd_z  UseExternalDerivativeSource=off  N=N_d  UseFilter=on  TunerSelectOption=Transfer Function Based (PID Tuner App)  InitialConditionSource=internal  InitialConditionForIntegrator=0  InitialConditionForFilter=0  DifferentiatorICPrevScaledInput=0  ExternalReset=none  TrackingMode=off  Kt=1  LimitOutput=on  SatLimitsSource=internal  UpperSaturationLimit=PID_LIMIT_Z+100  LowerSaturationLimit=-400  LinearizeAsGain=on  AntiWindupMode=clamping  Kb=1  LimitIntegrator=off  UpperIntegratorSaturationLimit=inf  LowerIntegratorSaturationLimit=-inf  POutMin=[]  POutMax=[]  IOutMin=[]  IOutMax=[]  DOutMin=[]  DOutMax=[]  NOutMin=[]  NOutMax=[]  SumOutMin=[]  SumOutMax=[]  SaturationOutMin=[]  SaturationOutMax=[]  PParamMin=[]  PParamMax=[]  IParamMin=[]  IParamMax=[]  DParamMin=[]  DParamMax=[]  NParamMin=[]  NParamMax=[]  KbParamMin=[]  KbParamMax=[]  KtParamMin=[]  KtParamMax=[]  KbOutMin=[]  KbOutMax=[]  KtOutMin=[]  KtOutMax=[]  IntegratorOutMin=[]  IntegratorOutMax=[]  FilterOutMin=[]  FilterOutMax=[]  SumI1OutMin=[]  SumI1OutMax=[]  SumI2OutMin=[]  SumI2OutMax=[]  SumI3OutMin=[]  SumI3OutMax=[]  SumI4OutMin=[]  SumI4OutMax=[]  SumDOutMin=[]  SumDOutMax=[]  DifferentiatorOutMin=[]  DifferentiatorOutMax=[]  FilterDiffOutCoefMin=[]  FilterDiffOutCoefMax=[]  ReciprocalOutMin=[]  ReciprocalOutMax=[]  SumDenOutMin=[]  SumDenOutMax=[]  SumNumOutMin=[]  SumNumOutMax=[]  DivideOutMin=[]  DivideOutMax=[]  UdiffTsProdOutMin=[]  UdiffTsProdOutMax=[]  NTsProdOutMin=[]  NTsProdOutMax=[]  UintegralTsProdOutMin=[]  UintegralTsProdOutMax=[]  UngainTsProdOutMin=[]  UngainTsProdOutMax=[]  ClampingZeroOutDataTypeStr=Inherit: Inherit via back propagation  ClampingZeroOutMin=[]  ClampingZeroOutMax=[]  FilterDenConstantOutDataTypeStr=Inherit: Inherit via back propagation  FilterDenConstantOutMin=[]  FilterDenConstantOutMax=[]  PCopyOutDataTypeStr=Inherit: Inherit via back propagation  PCopyOutMin=[]  PCopyOutMax=[]  NCopyOutDataTypeStr=Inherit: Inherit via back propagation  NCopyOutMin=[]  NCopyOutMax=[]  IntegratorContinuousStateAttributes=''  IntegratorStateMustResolveToSignalObject=off  IntegratorRTWStateStorageClass=Auto  FilterContinuousStateAttributes=''  FilterStateMustResolveToSignalObject=off  FilterRTWStateStorageClass=Auto  ParallelPVariant=InternalParameters  IdealPVariant=Disabled  IVariant=InternalParameters  DVariant=InternalParameters  IntegratorVariant=Continuous  SatVariant=Enabled  AWVariant=ContClampingParallel  PCopyVariant=Disabled  TRVariant=Disabled  FdbkBlocksVariant=Forward  IdealPFdbkVariant=Disabled  SatFdbkVariant=Disabled  DerivativeFilterVariant=ContFilter  NVariant=InternalParameters  NCopyVariant=Disabled  FilterICVariant=InternalICsFilter  IntegratorICVariant=InternalICs  ExternalResetVariant=Disabled  TRSumVariant=Passthrough  SumFdbkVariant=Disabled  SumVariant=Sum_PID  TsampFilterVariant=InternalTs  TsampNgainVariant=Passthrough  TsampIntegralVariant=Disabled_SignalSpec  ExternalSaturationOutDataTypeStr=Inherit: Same as second input  DerivativeSourceVariant=ErrorSignal  PreIntVariant=InternalPreInt
  u_roll : Outport
  u_pitch : Outport  Port=2
  u_yaw : Outport  Port=3
  u_z : Outport  Port=4
  wires:
  PID Controller10/1 -> u_roll/1  "u_roll"
  e_Yaw/1 -> PID Controller12/1
  PID Controller13/1 -> u_z/1  "u_z"
  e_Pitch/1 -> PID Controller11/1
  PID Controller12/1 -> u_yaw/1  "u_yaw"
  e_z/1 -> PID Controller13/1
  PID Controller11/1 -> u_pitch/1  "u_pitch"
  e_Roll/1 -> PID Controller10/1

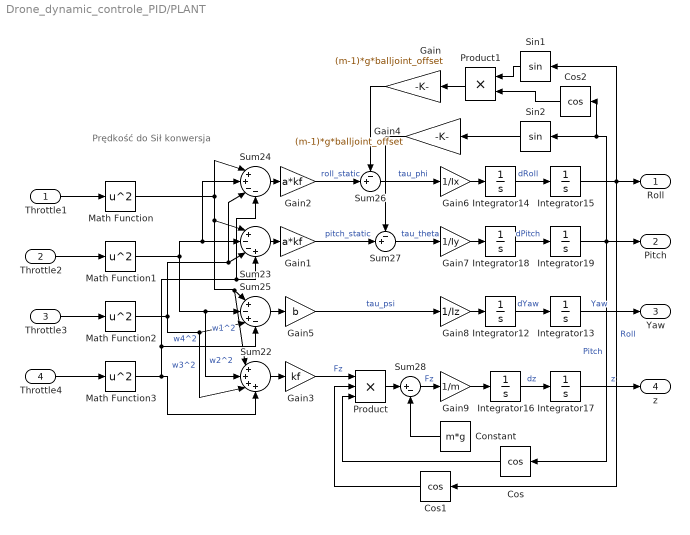
== system Drone_dynamic_controle_PID/PLANT ==
  note: Prędkość do Sił konwersja
  Throttle1 : Inport
  Throttle2 : Inport  Port=2
  Throttle3 : Inport  Port=3
  Throttle4 : Inport  Port=4
  Constant : Constant  Value=m*g
  Cos : Trigonometry  Operator=cos
  Cos1 : Trigonometry  Operator=cos
  Cos2 : Trigonometry  Operator=cos
  Gain : Gain  Gain=(m-1)*g*balljoint_offset
  Gain1 : Gain  Gain=a*kf
  Gain2 : Gain  Gain=a*kf
  Gain3 : Gain  Gain=kf
  Gain4 : Gain  Gain=(m-1)*g*balljoint_offset
  Gain5 : Gain  Gain=b
  Gain6 : Gain  Gain=1/Ix
  Gain7 : Gain  Gain=1/Iy
  Gain8 : Gain  Gain=1/Iz
  Gain9 : Gain  Gain=1/m
  Integrator{12..19} (8 alike) : Integrator
  Math Function{,1..3} (4 alike) : Math  Operator=square
  Product : Product  Inputs=3
  Product1 : Product
  Sin1 : Trigonometry
  Sin2 : Trigonometry
  Sum22 : Sum  Inputs=|++++
  Sum23 : Sum  Inputs=|+--+
  Sum24 : Sum  Inputs=|++--
  Sum25 : Sum  Inputs=|+-+-
  Sum26 : Sum  Inputs=-+|
  Sum27 : Sum  Inputs=-+|
  Sum28 : Sum  Inputs=|+-
  Roll : Outport
  Pitch : Outport  Port=2
  Yaw : Outport  Port=3
  z : Outport  Port=4
  wires:
  Integrator17/1 -> z/1  "z"
  Integrator12/1 -> Integrator13/1  "dYaw"
  Sum28/1 -> Gain9/1  "Fz"
  Product/1 -> Sum28/1
  Gain9/1 -> Integrator16/1
  Product1/1 -> Gain/1
  Integrator14/1 -> Integrator15/1  "dRoll"
  Sum26/1 -> Gain6/1  "tau_phi"
  Gain7/1 -> Integrator18/1
  Sum27/1 -> Gain7/1  "tau_theta"
  Gain4/1 -> Sum27/1
  Integrator13/1 -> Yaw/1  "Yaw"
  Cos/1 -> Product/3
  Integrator16/1 -> Integrator17/1  "dz"
  Cos1/1 -> Product/2
  Constant/1 -> Sum28/2
  Integrator18/1 -> Integrator19/1  "dPitch"
  Integrator15/1 -> Sin1/1, Roll/1, Cos1/1  "Roll"
  Gain/1 -> Sum26/1
  Cos2/1 -> Product1/2
  Gain8/1 -> Integrator12/1
  Gain6/1 -> Integrator14/1
  Integrator19/1 -> Cos/1, Pitch/1, Cos2/1, Sin2/1  "Pitch"
  Sin1/1 -> Product1/1
  Sin2/1 -> Gain4/1
  Gain2/1 -> Sum26/2  "roll_static"
  Throttle3/1 -> Math Function2/1
  Gain5/1 -> Gain8/1  "tau_psi"
  Math Function1/1 -> Sum22/2, Sum25/2, Sum23/2, Sum24/2  "w2^2"
  Gain3/1 -> Product/1  "Fz"
  Sum23/1 -> Gain1/1
  Sum24/1 -> Gain2/1
  Sum25/1 -> Gain5/1
  Throttle1/1 -> Math Function/1
  Throttle4/1 -> Math Function3/1
  Throttle2/1 -> Math Function1/1
  Sum22/1 -> Gain3/1
  Math Function/1 -> Sum22/1, Sum25/1, Sum23/1, Sum24/1  "w1^2"
  Math Function3/1 -> Sum22/4, Sum25/4, Sum23/4, Sum24/4  "w4^2"
  Gain1/1 -> Sum27/2  "pitch_static"
  Math Function2/1 -> Sum24/3, Sum23/3, Sum22/3, Sum25/3  "w3^2"

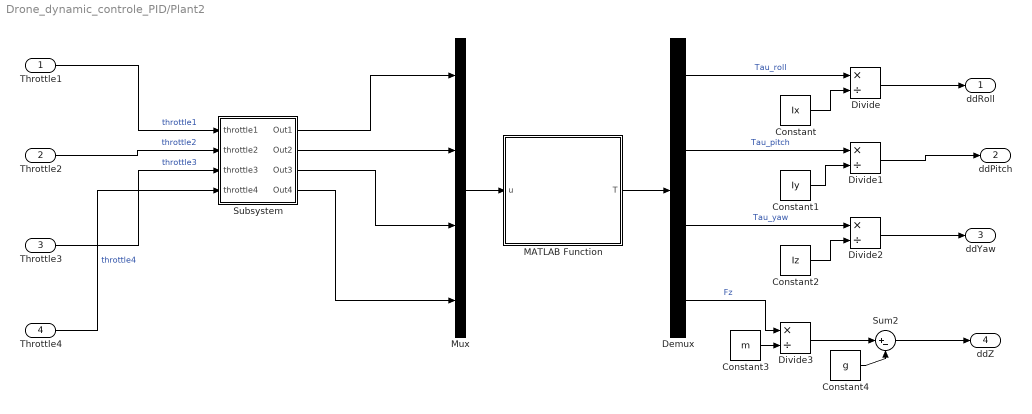
== system Drone_dynamic_controle_PID/Plant2 ==
  Throttle1 : Inport
  Throttle2 : Inport  Port=2
  Throttle3 : Inport  Port=3
  Throttle4 : Inport  Port=4
  Constant : Constant  Value=Ix
  Constant1 : Constant  Value=Iy
  Constant2 : Constant  Value=Iz
  Constant3 : Constant  Value=m
  Constant4 : Constant  Value=g
  Demux : Demux
  Divide{,1..3} (4 alike) : Product  Inputs=*/
  MATLAB Function : MATLAB Function  TreatAsAtomicUnit=on
  Mux : Mux
  Subsystem : Subsystem
  Sum2 : Sum  Inputs=|+-
  ddRoll : Outport
  ddPitch : Outport  Port=2
  ddYaw : Outport  Port=3
  ddZ : Outport  Port=4
  wires:
  Constant/1 -> Divide/2
  Constant4/1 -> Sum2/2
  Divide3/1 -> Sum2/1
  Constant1/1 -> Divide1/2
  Constant2/1 -> Divide2/2
  Demux/2 -> Divide1/1  "Tau_pitch"
  Constant3/1 -> Divide3/2
  Demux/1 -> Divide/1  "Tau_roll"
  Demux/3 -> Divide2/1  "Tau_yaw"
  Sum2/1 -> ddZ/1
  Divide2/1 -> ddYaw/1
  Demux/4 -> Divide3/1  "Fz"
  Divide1/1 -> ddPitch/1
  Divide/1 -> ddRoll/1
  MATLAB Function/1(T) -> Demux/1
  Mux/1 -> MATLAB Function/1(u)
  Throttle1/1 -> Subsystem/1(throttle1)  "throttle1"
  Throttle2/1 -> Subsystem/2(throttle2)  "throttle2"
  Throttle3/1 -> Subsystem/3(throttle3)  "throttle3"
  Throttle4/1 -> Subsystem/4(throttle4)  "throttle4"
  Subsystem/1(Out1) -> Mux/1
  Subsystem/2(Out2) -> Mux/2
  Subsystem/3(Out3) -> Mux/3
  Subsystem/4(Out4) -> Mux/4

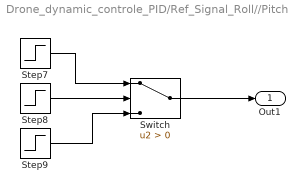
== system Drone_dynamic_controle_PID/Ref_Signal_Roll//Pitch ==
  Step7 : Step  Time=5  After=10  SampleTime=0.01
  Step8 : Step  Time=10  Before=1  After=0  SampleTime=0.01
  Step9 : Step  Time=15  Before=-10  After=0  SampleTime=0.01
  Switch : Switch  Criteria=u2 > Threshold  SaturateOnIntegerOverflow=off  InputSameDT=off
  Out1 : Outport
  wires:
  Step9/1 -> Switch/3
  Step8/1 -> Switch/2
  Step7/1 -> Switch/1
  Switch/1 -> Out1/1

== system Drone_dynamic_controle_PID/Ref_Signal_Yaw ==
  Step6 : Step  Time=15  Before=1  After=0  SampleTime=0.01
  Step7 : Step  Time=10  Before=100  After=200  SampleTime=0.01
  Step8 : Step  Time=15  Before=100  After=100  SampleTime=0.01
  Switch1 : Switch  Criteria=u2 > Threshold  SaturateOnIntegerOverflow=off  InputSameDT=off
  Out1 : Outport
  wires:
  Step7/1 -> Switch1/1
  Step6/1 -> Switch1/2
  Step8/1 -> Switch1/3
  Switch1/1 -> Out1/1

== system Drone_dynamic_controle_PID/Ref_Signal_Z ==
  Step10 : Step  Time=10  Before=10  After=20  SampleTime=0.01
  Step6 : Step  Time=15  Before=10  After=10  SampleTime=0.01
  Step7 : Step  Time=15  Before=1  After=0  SampleTime=0.01
  Switch2 : Switch  Criteria=u2 > Threshold  SaturateOnIntegerOverflow=off  InputSameDT=off
  Out1 : Outport
  wires:
  Step7/1 -> Switch2/2
  Step10/1 -> Switch2/1
  Step6/1 -> Switch2/3
  Switch2/1 -> Out1/1

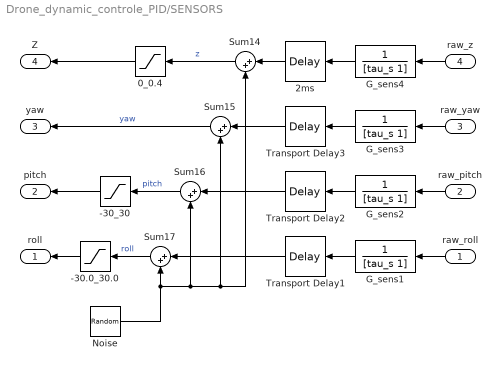
== system Drone_dynamic_controle_PID/SENSORS ==
  raw_roll : Inport
  raw_pitch : Inport  Port=2
  raw_yaw : Inport  Port=3
  raw_z : Inport  Port=4
  -30.0_30.0 : Saturate  UpperLimit=40  LowerLimit=0
  -30_30 : Saturate  UpperLimit=40  LowerLimit=0
  0_0.4 : Saturate  UpperLimit=40  LowerLimit=0
  2ms : TransportDelay  DelayTime=0.002
  G_sens{1..4} (4 alike) : TransferFcn  Denominator=[tau_s 1]
  Noise : RandomNumber  Variance=0.000025  Seed=12345  SampleTime=0.01
  Sum{14..17} (4 alike) : Sum  Inputs=|++
  Transport Delay1 : TransportDelay  DelayTime=0.002
  Transport Delay2 : TransportDelay  DelayTime=0.002
  Transport Delay3 : TransportDelay  DelayTime=0.002
  roll : Outport
  pitch : Outport  Port=2
  yaw : Outport  Port=3
  Z : Outport  Port=4
  wires:
  Sum14/1 -> 0_0.4/1  "z"
  Sum16/1 -> -30_30/1  "pitch"
  Transport Delay1/1 -> Sum17/1
  Noise/1 -> Sum14/2, Sum15/2, Sum16/2, Sum17/2
  G_sens1/1 -> Transport Delay1/1
  Transport Delay2/1 -> Sum16/1
  raw_pitch/1 -> G_sens2/1
  Transport Delay3/1 -> Sum15/1
  0_0.4/1 -> Z/1
  G_sens4/1 -> 2ms/1
  G_sens3/1 -> Transport Delay3/1
  G_sens2/1 -> Transport Delay2/1
  2ms/1 -> Sum14/1
  Sum15/1 -> yaw/1  "yaw"
  Sum17/1 -> -30.0_30.0/1  "roll"
  raw_yaw/1 -> G_sens3/1
  raw_z/1 -> G_sens4/1
  raw_roll/1 -> G_sens1/1
  -30_30/1 -> pitch/1
  -30.0_30.0/1 -> roll/1

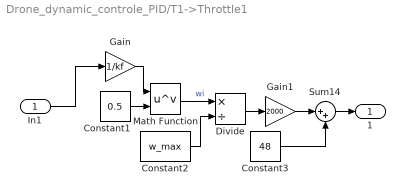
== system Drone_dynamic_controle_PID/T1->Throttle1 ==
  In1 : Inport
  Constant1 : Constant  Value=0.5
  Constant2 : Constant  Value=w_max
  Constant3 : Constant  Value=48
  Divide : Product  Inputs=*/
  Gain : Gain  Gain=1/kf
  Gain1 : Gain  Gain=2000
  Math Function : Math  Operator=pow
  Sum14 : Sum  Inputs=|++
  1 : Outport
  wires:
  Constant3/1 -> Sum14/2
  Gain/1 -> Math Function/1
  Sum14/1 -> 1/1
  Gain1/1 -> Sum14/1
  Math Function/1 -> Divide/1  "wi"
  In1/1 -> Gain/1
  Constant2/1 -> Divide/2
  Constant1/1 -> Math Function/2
  Divide/1 -> Gain1/1

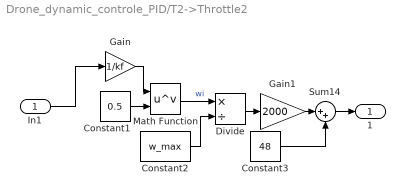
== system Drone_dynamic_controle_PID/T2->Throttle2 ==
  In1 : Inport
  Constant1 : Constant  Value=0.5
  Constant2 : Constant  Value=w_max
  Constant3 : Constant  Value=48
  Divide : Product  Inputs=*/
  Gain : Gain  Gain=1/kf
  Gain1 : Gain  Gain=2000
  Math Function : Math  Operator=pow  OutputSignalType=real
  Sum14 : Sum  Inputs=|++
  1 : Outport
  wires:
  Constant3/1 -> Sum14/2
  Gain/1 -> Math Function/1
  Sum14/1 -> 1/1
  Gain1/1 -> Sum14/1
  Math Function/1 -> Divide/1  "wi"
  In1/1 -> Gain/1
  Constant2/1 -> Divide/2
  Constant1/1 -> Math Function/2
  Divide/1 -> Gain1/1

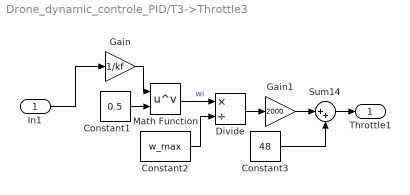
== system Drone_dynamic_controle_PID/T3->Throttle3 ==
  In1 : Inport
  Constant1 : Constant  Value=0.5
  Constant2 : Constant  Value=w_max
  Constant3 : Constant  Value=48
  Divide : Product  Inputs=*/
  Gain : Gain  Gain=1/kf
  Gain1 : Gain  Gain=2000
  Math Function : Math  Operator=pow
  Sum14 : Sum  Inputs=|++
  Throttle1 : Outport
  wires:
  Constant3/1 -> Sum14/2
  Gain/1 -> Math Function/1
  Sum14/1 -> Throttle1/1
  Gain1/1 -> Sum14/1
  Math Function/1 -> Divide/1  "wi"
  In1/1 -> Gain/1
  Constant2/1 -> Divide/2
  Constant1/1 -> Math Function/2
  Divide/1 -> Gain1/1

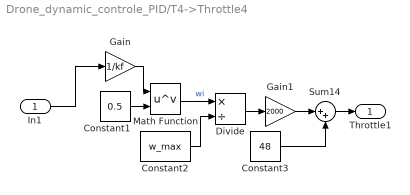
== system Drone_dynamic_controle_PID/T4->Throttle4 ==
  In1 : Inport
  Constant1 : Constant  Value=0.5
  Constant2 : Constant  Value=w_max
  Constant3 : Constant  Value=48
  Divide : Product  Inputs=*/
  Gain : Gain  Gain=1/kf
  Gain1 : Gain  Gain=2000
  Math Function : Math  Operator=pow
  Sum14 : Sum  Inputs=|++
  Throttle1 : Outport
  wires:
  Constant3/1 -> Sum14/2
  Gain/1 -> Math Function/1
  Sum14/1 -> Throttle1/1
  Gain1/1 -> Sum14/1
  Math Function/1 -> Divide/1  "wi"
  In1/1 -> Gain/1
  Constant2/1 -> Divide/2
  Constant1/1 -> Math Function/2
  Divide/1 -> Gain1/1

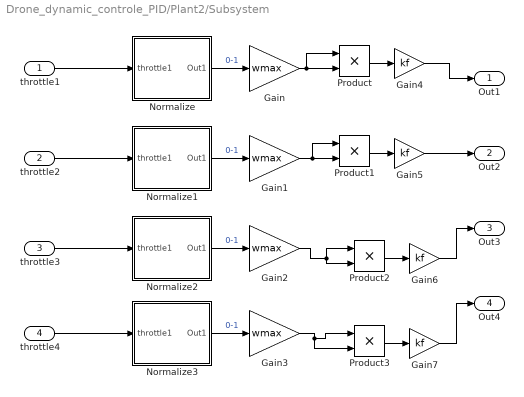
== system Drone_dynamic_controle_PID/Plant2/Subsystem ==
  throttle1 : Inport
  throttle2 : Inport  Port=2
  throttle3 : Inport  Port=3
  throttle4 : Inport  Port=4
  Gain{,1..3} (4 alike) : Gain  Gain=wmax
  Gain{4..7} (4 alike) : Gain  Gain=kf
  Normalize : Subsystem
  Normalize1 : Subsystem
  Normalize2 : Subsystem
  Normalize3 : Subsystem
  Product{,1..3} (4 alike) : Product
  Out1 : Outport
  Out2 : Outport  Port=2
  Out3 : Outport  Port=3
  Out4 : Outport  Port=4
  wires:
  Product1/1 -> Gain5/1
  Gain/1 -> Product/1, Product/2
  Normalize/1(Out1) -> Gain/1  "0-1"
  throttle2/1 -> Normalize1/1(throttle1)
  Normalize3/1(Out1) -> Gain3/1  "0-1"
  Normalize2/1(Out1) -> Gain2/1  "0-1"
  Normalize1/1(Out1) -> Gain1/1  "0-1"
  Gain5/1 -> Out2/1
  Gain3/1 -> Product3/2, Product3/1
  Product2/1 -> Gain6/1
  Product3/1 -> Gain7/1
  Gain2/1 -> Product2/1, Product2/2
  Product/1 -> Gain4/1
  Gain1/1 -> Product1/2, Product1/1
  throttle1/1 -> Normalize/1(throttle1)
  throttle3/1 -> Normalize2/1(throttle1)
  throttle4/1 -> Normalize3/1(throttle1)
  Gain4/1 -> Out1/1
  Gain7/1 -> Out4/1
  Gain6/1 -> Out3/1

== system Drone_dynamic_controle_PID/Plant2/Subsystem/Normalize ==
  throttle1 : Inport
  Constant5 : Constant  Value=48
  Multiply : Gain  Gain=1/2000
  Sum : Sum  Inputs=|+-
  Out1 : Outport
  wires:
  Sum/1 -> Multiply/1
  Constant5/1 -> Sum/2
  throttle1/1 -> Sum/1
  Multiply/1 -> Out1/1

== system Drone_dynamic_controle_PID/Plant2/Subsystem/Normalize1 ==
  throttle1 : Inport
  Constant5 : Constant  Value=48
  Multiply : Gain  Gain=1/2000
  Sum : Sum  Inputs=|+-
  Out1 : Outport
  wires:
  Sum/1 -> Multiply/1
  Constant5/1 -> Sum/2
  throttle1/1 -> Sum/1
  Multiply/1 -> Out1/1

== system Drone_dynamic_controle_PID/Plant2/Subsystem/Normalize2 ==
  throttle1 : Inport
  Constant5 : Constant  Value=48
  Multiply : Gain  Gain=1/2000
  Sum : Sum  Inputs=|+-
  Out1 : Outport
  wires:
  Sum/1 -> Multiply/1
  Constant5/1 -> Sum/2
  throttle1/1 -> Sum/1
  Multiply/1 -> Out1/1

== system Drone_dynamic_controle_PID/Plant2/Subsystem/Normalize3 ==
  throttle1 : Inport
  Constant5 : Constant  Value=48
  Multiply : Gain  Gain=1/2000
  Sum : Sum  Inputs=|+-
  Out1 : Outport
  wires:
  Sum/1 -> Multiply/1
  Constant5/1 -> Sum/2
  throttle1/1 -> Sum/1
  Multiply/1 -> Out1/1

== matlab function Drone_dynamic_controle_PID/Plant2/MATLAB Function ==
  data: u input; T output
function T = mixer(u)
% u = [T1; T2; T3; T4]

    % Parametry
    L = 0.25;           % długość ramienia [m]
    kf = 6.11e-8;       % współczynnik siły
    km = 1.5e-9;        % współczynnik momentu

    % Macierz miksera
    M = [ L/sqrt(2), -L/sqrt(2), -L/sqrt(2),  L/sqrt(2);
          L/sqrt(2),  L/sqrt(2), -L/sqrt(2), -L/sqrt(2);
               km,        -km,       km,       -km;
               kf,         kf,       kf,        kf ];

    % Odwrotność i obliczenie T
    T = M * u;
end

== matlab function Drone_dynamic_controle_PID/MATLAB Function ==
  data: u input; T output
function T = inverse_mixer(u)
% u = [tau_phi; tau_theta; tau_psi; Fz]

    % Parametry
    l  = 0.2;
    kf=1.228775212611820e-04;
    km = 1.5e-9;

    % Macierz miksera
    M = [ l/sqrt(2), -l/sqrt(2), -l/sqrt(2),  l/sqrt(2);
          l/sqrt(2),  l/sqrt(2), -l/sqrt(2), -l/sqrt(2);
               km,        -km,       km,       -km;
               kf,         kf,       kf,        kf ];

    % Odwrotność i obliczenie T
    T = inv(M) * u;
end
